simulink model "zumo_control_distance_heading"  (R2014a)
settings: Solver=ode3  SolverMode=SingleTasking  StartTime=0.0  StopTime=10  FixedStep=0.01  RelTol=1e-3
PreLoadFcn:
  | evalin('base','sim=1;');
  | evalin('base','control=0;');
  | prepareCurrentFolderForZumo;
  | load MagnetometerBus;
model workspace (MAT data in the model file):
  axleLength = Simulink.Parameter
  axleLength.Value = 9.8
  axleLength.Description = 'Distance between tire contact points
    | of the two wheels/treads
    | in units of centimeters.'
  axleLength.DataType = 'auto'
  commandPercmPerSecond = Simulink.Parameter
  commandPercmPerSecond.Value = 3.9547
  commandPercmPerSecond.Description = 'Convert units of ''command'' 
    | to units of ''cm/s''.
    | 
    | ''command'' is a value in the range [-256, 255].'
  commandPercmPerSecond.DataType = 'auto'
  symmetrizeMotors = Simulink.Parameter
  symmetrizeMotors.Value = 1
  symmetrizeMotors.Description = 'Scale one of the motor commands down 
    | (not up) to balance the motors. 
    | Once balanced, a value of x sent to either
    | motor will produce the same rate of rotation
    | in both motors.'
  symmetrizeMotors.DataType = 'auto'
  sampleTime = Simulink.Parameter
  sampleTime.Value = 0.01
  sampleTime.Description = 'Sample time (in seconds) of the trajectory simulator.'
  sampleTime.DataType = 'auto'
  commandThreshold = Simulink.Parameter
  commandThreshold.Value = 31.875
  commandThreshold.DataType = 'auto'
  lineThreshold = Simulink.Parameter
  lineThreshold.Value = 500
  lineThreshold.DataType = 'auto'
  velocity = Simulink.Parameter
  velocity.Value = 10
  velocity.Description = 'cm / s'
  velocity.DataType = 'auto'
  waveLength = Simulink.Parameter
  waveLength.Value = 8.6
  waveLength.Description = 'Units of cm.
    | 
    | The following condition must be satisfied: 
    | waveLength > 2*pi * velocity / sqrt(0.5 / sampleTime)
    | 
    | For reference,
    | robotLength = 8.6 cm
    | '
  waveLength.DataType = 'auto'
  compassBias = Simulink.Parameter
  compassBias.Value = 0
  compassBias.DataType = 'auto'
undefined symbols (not defined in the file or in its folder): DiscIntNeverNeededParam, magnitude
libraries: simulink x2, ZumoBotLib x2
settings Model: ExtModeTrigDuration=2  Creator=pkasseba  LastModifiedBy=sandip
settings OptimizationCC: OptimizeModelRefInitCode=on  LifeSpan=1
settings DebuggingCC: UnderspecifiedInitializationDetection=Classic  SolverPrmCheckMsg=none  StateNameClashWarn=warning
settings HardwareCC: ProdBitPerInt=16  ProdBitPerPointer=8  ProdIntDivRoundTo=Zero  ProdEndianess=LittleEndian  ProdWordSize=8  ProdHWDeviceType=Atmel->AVR
settings SFSimCC: SimParseCustomCode=off
settings RTWCC: SystemTargetFile=realtime.tlc  GenerateMakefile=off  TemplateMakefile=realtime.tmf  Description=Run on Target Hardware  RTWVerbose=off  ProcessScript=realtime_make_rtw_hook
settings STFCustomTargetCC: TargetLibSuffix=.a  GenerateSampleERTMain=on  ConcurrentExecutionCompliant=off  GeneratePreprocessorConditionals=Use local settings  ERTCustomFileBanners=on  SupportNonInlinedSFcns=off  SupportVariableSizeSignals=on  MATLABClassNameForMDSCustomization=Simulink.SoftwareTarget.ERTCustomization  GRTInterface=off  SystemTargetFile=realtime.tlc
settings ERTTargetCC: CombineOutputUpdateFcns=off  SupportContinuousTime=on  SupportVariableSizeSignals=on  ExtModeTransport=3  ExtModeMexFile=ext_serial_win32_comm  ExtModeMexArgs=0 1 9600  ERTSrcFileBannerTemplate=realtime_code_template.cgt  ERTHdrFileBannerTemplate=realtime_code_template.cgt  ERTDataSrcFileTemplate=realtime_code_template.cgt  ERTDataHdrFileTemplate=realtime_code_template.cgt  ERTCustomFileTemplate=realtime_file_process.tlc

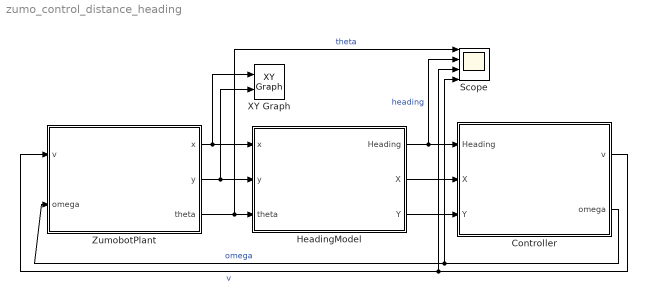
== system zumo_control_distance_heading ==
  Controller : Subsystem
  HeadingModel : Subsystem  Variant=on
  Scope : Scope  NumInputPorts=4
      settings: TimeRange=10  YMin=0~30.4~-1500~-5  YMax=375~33.6~1750~5  SaveName=ScopeData4
  XY Graph : simulink/Sinks/XY Graph  xmin=-20  xmax=20  ymin=-20  ymax=20  st=-1
  ZumobotPlant : Subsystem  Variant=on
  wires:
  Controller/1(v) -> Scope/3, ZumobotPlant/1(v)  "v"
  ZumobotPlant/1(x) -> XY Graph/1, HeadingModel/1(x)
  ZumobotPlant/2(y) -> XY Graph/2, HeadingModel/2(y)
  HeadingModel/1(Heading) -> Scope/2, Controller/1(Heading)  "heading"
  Controller/2(omega) -> Scope/4, ZumobotPlant/2(omega)  "omega"
  ZumobotPlant/3(theta) -> Scope/1, HeadingModel/3(theta)  "theta"
  HeadingModel/2(X) -> Controller/2(X)
  HeadingModel/3(Y) -> Controller/3(Y)

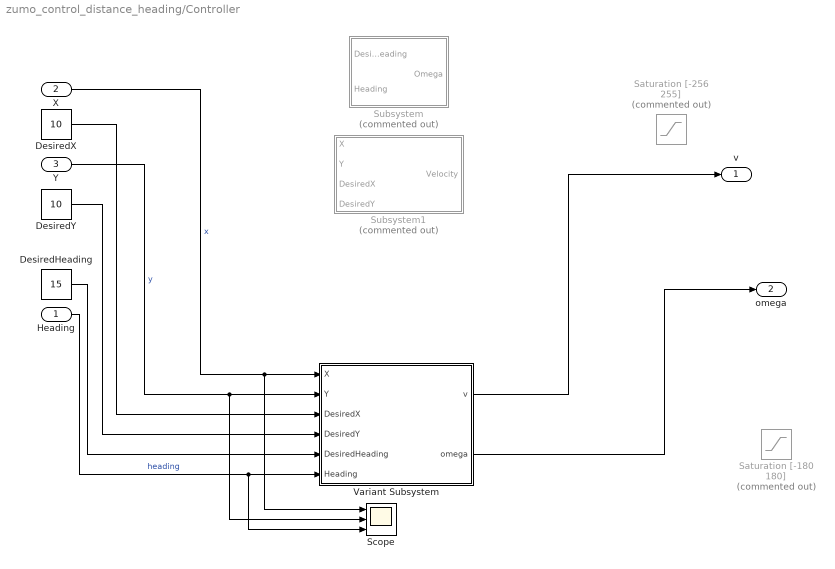
== system zumo_control_distance_heading/Controller ==
  Heading : Inport
  X : Inport  Port=2
  Y : Inport  Port=3
  DesiredHeading : Constant  Value=15
  DesiredX : Constant  Value=10
  DesiredY : Constant  Value=10
  Saturation [-180 180] : Saturate  Commented=on  UpperLimit=180  LowerLimit=-180
  Saturation [-256 255] : Saturate  Commented=on  UpperLimit=255  LowerLimit=-256
  Scope : Scope  NumInputPorts=3
      settings: YMin=0~-3~0  YMax=20~4~400  SaveName=ScopeData2
  Subsystem : Subsystem  Commented=on
  Subsystem1 : Subsystem  Commented=on
  Variant Subsystem : Subsystem  Variant=on  OverrideUsingVariant=control==0
  v : Outport
  omega : Outport  Port=2
  wires:
  X/1 -> Variant Subsystem/1(X), Scope/1  "x"
  Y/1 -> Variant Subsystem/2(Y), Scope/2  "y"
  DesiredX/1 -> Variant Subsystem/3(DesiredX)
  DesiredY/1 -> Variant Subsystem/4(DesiredY)
  DesiredHeading/1 -> Variant Subsystem/5(DesiredHeading)
  Heading/1 -> Variant Subsystem/6(Heading), Scope/3  "heading"
  Variant Subsystem/1(v) -> v/1
  Variant Subsystem/2(omega) -> omega/1

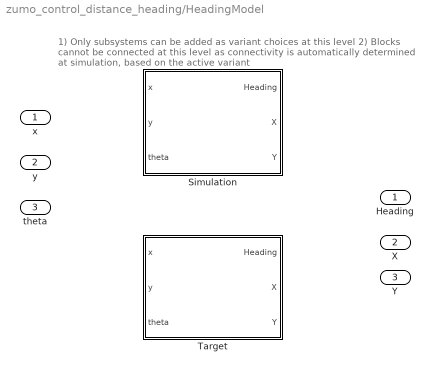
== system zumo_control_distance_heading/HeadingModel ==
  note: 1) Only subsystems can be added as variant choices at this level
      | 2) Blocks cannot be connected at this level as connectivity is
      | automatically determined at simulation, based on the active variant
  x : Inport
  y : Inport  Port=2
  theta : Inport  Port=3
  Simulation : Subsystem  VariantControl=sim==1
  Target : Subsystem  VariantControl=sim==0
  Heading : Outport
  X : Outport  Port=2
  Y : Outport  Port=3

== system zumo_control_distance_heading/ZumobotPlant ==
  note: 1) Only subsystems can be added as variant choices at this level
      | 2) Blocks cannot be connected at this level as connectivity is
      | automatically determined at simulation, based on the active variant
  v : Inport
  omega : Inport  Port=2
  Simulation : Subsystem  VariantControl=sim==1
  Target : Subsystem  VariantControl=sim==0
  x : Outport
  y : Outport  Port=2
  theta : Outport  Port=3

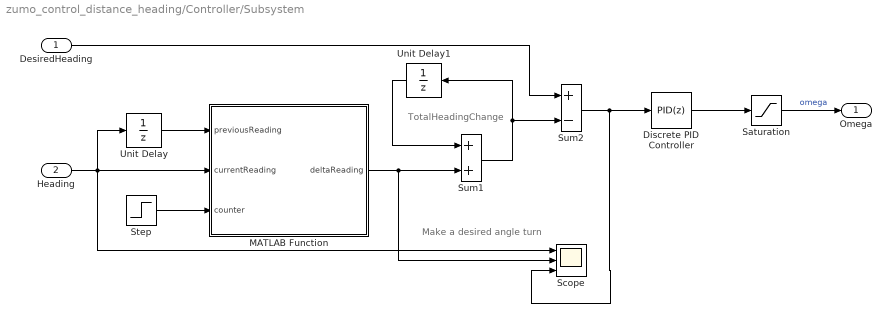
== system zumo_control_distance_heading/Controller/Subsystem ==
  note: Make a desired angle turn
  note: TotalHeadingChange
  DesiredHeading : Inport
  Heading : Inport  Port=2
  Discrete PID Controller : simulink/Continuous/PID Controller  Controller=PID  TimeDomain=Discrete-time  SampleTime=0.01  IntegratorMethod=Forward Euler  FilterMethod=Forward Euler  Form=Parallel  P=20  I=0  D=0  N=100  InitialConditionSource=internal  InitialConditionForIntegrator=0  InitialConditionForFilter=0  ExternalReset=none  LimitOutput=off  UpperSaturationLimit=inf  LowerSaturationLimit=-inf  LinearizeAsGain=off  AntiWindupMode=none  Kb=1  TrackingMode=off  Kt=1  PParamMin=[]  PParamMax=[]  IParamMin=[]  IParamMax=[]  DParamMin=[]  DParamMax=[]  NParamMin=[]  NParamMax=[]  KbParamMin=[]  KbParamMax=[]  KtParamMin=[]  KtParamMax=[]  POutMin=[]  POutMax=[]  IOutMin=[]  IOutMax=[]  DOutMin=[]  DOutMax=[]  NOutMin=[]  NOutMax=[]  KbOutMin=[]  KbOutMax=[]  KtOutMin=[]  KtOutMax=[]  IntegratorOutMin=[]  IntegratorOutMax=[]  FilterOutMin=[]  FilterOutMax=[]  SumOutMin=[]  SumOutMax=[]  SumI1OutMin=[]  SumI1OutMax=[]  SumI2OutMin=[]  SumI2OutMax=[]  SumI3OutMin=[]  SumI3OutMax=[]  SumDOutMin=[]  SumDOutMax=[]  SaturationOutMin=[]  SaturationOutMax=[]  IntegratorContinuousStateAttributes=''  IntegratorStateMustResolveToSignalObject=off  IntegratorRTWStateStorageClass=Auto  FilterContinuousStateAttributes=''  FilterStateMustResolveToSignalObject=off  FilterRTWStateStorageClass=Auto
  MATLAB Function : MATLAB Function  TreatAsAtomicUnit=on
  Saturation : Saturate  UpperLimit=200  LowerLimit=0
  Scope : Scope  NumInputPorts=3
      settings: YMin=266~-1~-4  YMax=266~1~-4
  Step : Step  Time=2*sampleTime  SampleTime=sampleTime
  Sum1 : Sum
  Sum2 : Sum  Inputs=+-
  Unit Delay : UnitDelay  SampleTime=-1
  Unit Delay1 : UnitDelay  SampleTime=-1
  Omega : Outport
  wires:
  Sum1/1 -> Unit Delay1/1, Sum2/2
  Step/1 -> MATLAB Function/3(counter)
  MATLAB Function/1(deltaReading) -> Scope/2, Sum1/2
  Sum2/1 -> Discrete PID Controller/1, Scope/3
  Saturation/1 -> Omega/1  "omega"
  Unit Delay/1 -> MATLAB Function/1(previousReading)
  Unit Delay1/1 -> Sum1/1
  DesiredHeading/1 -> Sum2/1
  Heading/1 -> Unit Delay/1, MATLAB Function/2(currentReading), Scope/1
  Discrete PID Controller/1 -> Saturation/1

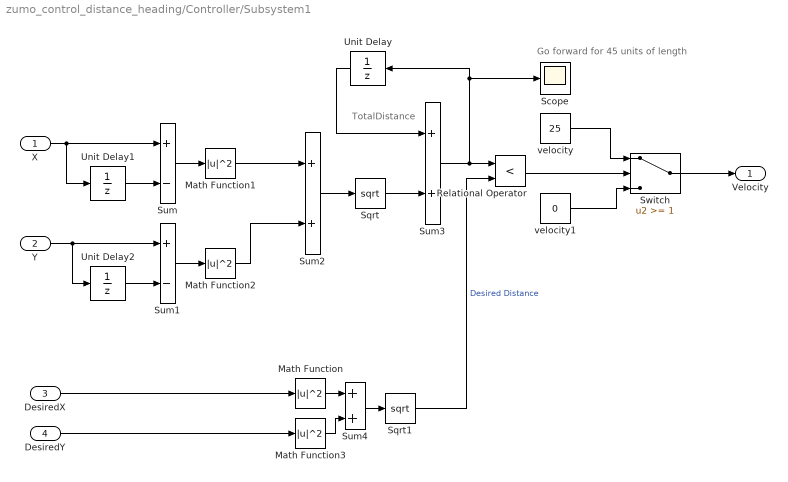
== system zumo_control_distance_heading/Controller/Subsystem1 ==
  note: Go forward for 45 units of length
  note: TotalDistance
  X : Inport
  Y : Inport  Port=2
  DesiredX : Inport  Port=3
  DesiredY : Inport  Port=4
  Math Function{,1..3} (4 alike) : Math  Operator=magnitude^2  SaturateOnIntegerOverflow=on
  Relational Operator : RelationalOperator  Operator=<  OutDataTypeStr=boolean
  Scope : Scope
      settings: YMin=0  YMax=50
  Sqrt : Sqrt  SaturateOnIntegerOverflow=on
  Sqrt1 : Sqrt  SaturateOnIntegerOverflow=on
  Sum : Sum  Inputs=+-
  Sum1 : Sum  Inputs=+-
  Sum2 : Sum
  Sum3 : Sum
  Sum4 : Sum
  Switch : Switch  Threshold=1
  Unit Delay : UnitDelay  SampleTime=-1
  Unit Delay1 : UnitDelay  SampleTime=-1
  Unit Delay2 : UnitDelay  SampleTime=-1
  velocity : Constant  Value=25
  velocity1 : Constant  Value=0
  Velocity : Outport
  wires:
  X/1 -> Unit Delay1/1, Sum/1
  Sqrt/1 -> Sum3/2
  Sum/1 -> Math Function1/1
  Sum2/1 -> Sqrt/1
  Math Function1/1 -> Sum2/1
  velocity/1 -> Switch/1
  Unit Delay1/1 -> Sum/2
  Math Function2/1 -> Sum2/2
  Switch/1 -> Velocity/1
  Sum1/1 -> Math Function2/1
  Unit Delay2/1 -> Sum1/2
  Y/1 -> Unit Delay2/1, Sum1/1
  Unit Delay/1 -> Sum3/1
  Sum3/1 -> Relational Operator/1, Scope/1, Unit Delay/1
  velocity1/1 -> Switch/3
  Relational Operator/1 -> Switch/2
  Math Function3/1 -> Sum4/2
  Math Function/1 -> Sum4/1
  Sum4/1 -> Sqrt1/1
  Sqrt1/1 -> Relational Operator/2  "Desired Distance"
  DesiredX/1 -> Math Function/1
  DesiredY/1 -> Math Function3/1

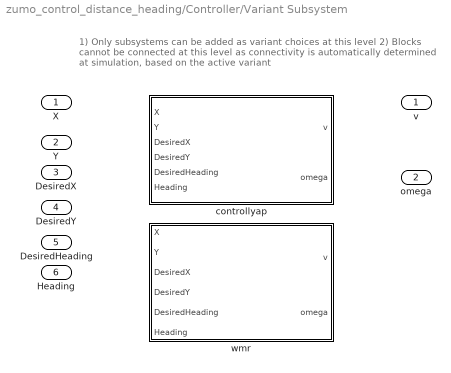
== system zumo_control_distance_heading/Controller/Variant Subsystem ==
  note: 1) Only subsystems can be added as variant choices at this level
      | 2) Blocks cannot be connected at this level as connectivity is
      | automatically determined at simulation, based on the active variant
  X : Inport
  Y : Inport  Port=2
  DesiredX : Inport  Port=3
  DesiredY : Inport  Port=4
  DesiredHeading : Inport  Port=5
  Heading : Inport  Port=6
  controllyap : MATLAB Function  TreatAsAtomicUnit=on  VariantControl=control==0
  wmr : MATLAB Function  TreatAsAtomicUnit=on  VariantControl=control==1
  v : Outport
  omega : Outport  Port=2

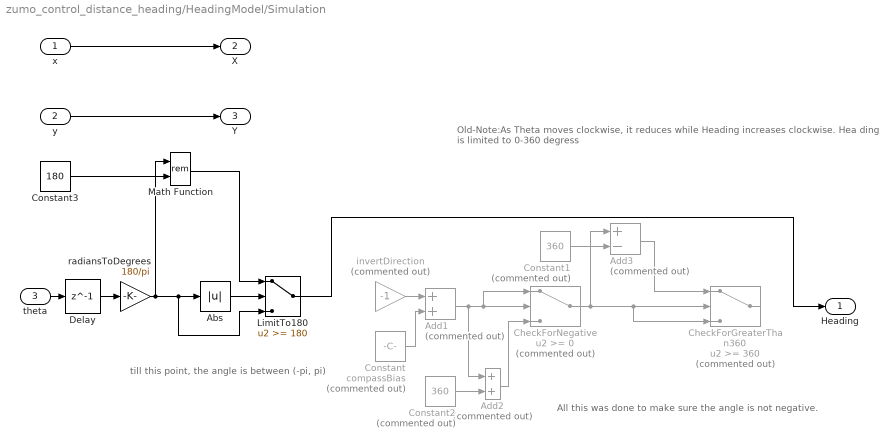
== system zumo_control_distance_heading/HeadingModel/Simulation ==
  note: till this point, the angle is between (-pi, pi)
  note: All this was done to make sure the angle is not negative.
  note: Old-Note:As Theta moves clockwise, it reduces while Heading increases clockwise.
      | Hea ding is limited to 0-360 degress
  x : Inport
  y : Inport  Port=2
  theta : Inport  Port=3
  Abs : Abs
  Add1 : Sum  Commented=on
  Add2 : Sum  Commented=on
  Add3 : Sum  Commented=on  Inputs=+-
  CheckForGreaterThan360 : Switch  Commented=on  Threshold=360
  CheckForNegative : Switch  Commented=on
  Constant : Constant  Commented=on  Value=compassBias
  Constant1 : Constant  Commented=on  Value=360
  Constant2 : Constant  Commented=on  Value=360
  Constant3 : Constant  Value=180
  Delay : Delay  DelayLength=1  InitialCondition=2*pi  SampleTime=sampleTime
  LimitTo180 : Switch  Threshold=180
  Math Function : Math  Operator=rem  SaturateOnIntegerOverflow=on
  invertDirection : Gain  Commented=on  Gain=-1
  radiansToDegrees : Gain  Gain=180/pi
  Heading : Outport
  X : Outport  Port=2
  Y : Outport  Port=3
  wires:
  x/1 -> X/1
  y/1 -> Y/1
  theta/1 -> Delay/1
  Delay/1 -> radiansToDegrees/1
  Constant/1 -> Add1/2
  Constant1/1 -> Add3/2
  Add3/1 -> CheckForGreaterThan360/1
  invertDirection/1 -> Add1/1
  Add1/1 -> Add2/1, CheckForNegative/2, CheckForNegative/1
  CheckForNegative/1 -> CheckForGreaterThan360/3, CheckForGreaterThan360/2, Add3/1
  Constant2/1 -> Add2/2
  Add2/1 -> CheckForNegative/3
  radiansToDegrees/1 -> Math Function/1, LimitTo180/3, Abs/1
  Constant3/1 -> Math Function/2
  Math Function/1 -> LimitTo180/1
  Abs/1 -> LimitTo180/2
  LimitTo180/1 -> Heading/1

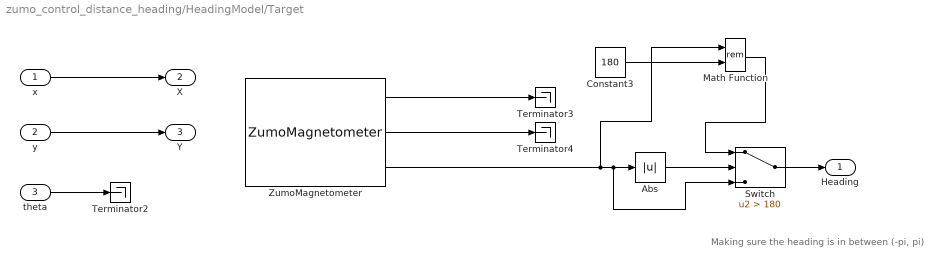
== system zumo_control_distance_heading/HeadingModel/Target ==
  note: Making sure the heading is in between (-pi, pi)
  x : Inport
  y : Inport  Port=2
  theta : Inport  Port=3
  Abs : Abs
  Constant3 : Constant  Value=180
  Math Function : Math  Operator=rem  SaturateOnIntegerOverflow=on
  Switch : Switch  Criteria=u2 > Threshold  Threshold=180
  Terminator2 : Terminator
  Terminator3 : Terminator
  Terminator4 : Terminator
  ZumoMagnetometer : ZumoBotLib/ZumoMagnetometer  sampletime_lsm=0.01  debug_lsm=on  minX_lsm=-512  maxX_lsm=-279  minY_lsm=-163  maxY_lsm=99  minZ_lsm=1302  maxZ_lsm=1580
      link override S-Function Builder: Parameters=sampletime_lsm,boolean(debug_lsm),minX_lsm,maxX_lsm,minY_lsm,maxY_lsm,minZ_lsm,boolean(maxZ_lsm)
  Heading : Outport
  X : Outport  Port=2
  Y : Outport  Port=3
  wires:
  x/1 -> X/1
  y/1 -> Y/1
  theta/1 -> Terminator2/1
  ZumoMagnetometer/1 -> Terminator3/1
  ZumoMagnetometer/2 -> Terminator4/1
  Switch/1 -> Heading/1
  Abs/1 -> Switch/2
  ZumoMagnetometer/3 -> Math Function/1, Switch/3, Abs/1
  Constant3/1 -> Math Function/2
  Math Function/1 -> Switch/1

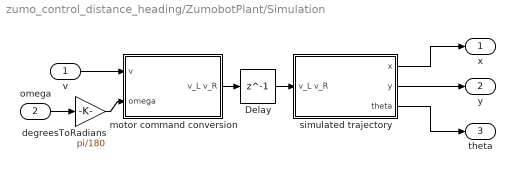
== system zumo_control_distance_heading/ZumobotPlant/Simulation ==
  v : Inport
  omega : Inport  Port=2
  Delay : Delay  DelayLength=1  InitialCondition=0
  degreesToRadians : Gain  Gain=pi/180
  motor command conversion : Subsystem
  simulated trajectory : Subsystem
  x : Outport
  y : Outport  Port=2
  theta : Outport  Port=3
  wires:
  v/1 -> motor command conversion/1(v)
  simulated trajectory/1(x) -> x/1
  simulated trajectory/2(y) -> y/1
  omega/1 -> degreesToRadians/1
  simulated trajectory/3(theta) -> theta/1
  degreesToRadians/1 -> motor command conversion/2(omega)
  motor command conversion/1(v_L v_R) -> Delay/1
  Delay/1 -> simulated trajectory/1(v_L v_R)

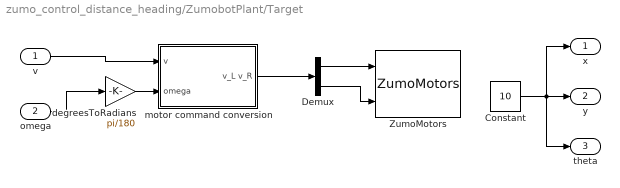
== system zumo_control_distance_heading/ZumobotPlant/Target ==
  v : Inport
  omega : Inport  Port=2
  Constant : Constant  Value=10
  Demux : Demux  Outputs=2
  ZumoMotors : ZumoBotLib/ZumoMotors  flipLeft=off  flipRight=off
  degreesToRadians : Gain  Gain=pi/180
  motor command conversion : Subsystem
  x : Outport
  y : Outport  Port=2
  theta : Outport  Port=3
  wires:
  motor command conversion/1(v_L v_R) -> Demux/1
  Demux/1 -> ZumoMotors/1
  Demux/2 -> ZumoMotors/2
  v/1 -> motor command conversion/1(v)
  Constant/1 -> theta/1, x/1, y/1
  omega/1 -> degreesToRadians/1
  degreesToRadians/1 -> motor command conversion/2(omega)

== system zumo_control_distance_heading/ZumobotPlant/Simulation/motor command conversion ==
  note: or in matrix notation,
  note: v_L  = v - omega * axleLength/2
      | v_R = v + omega * axleLength/2
  note: [v_L; v_R] = [1 -axleLength/2; 1 axleLength/2] * [v; omega]
  v : Inport
  omega : Inport  Port=2
  Mux : Mux  Inputs=2
  Saturation [-256 255] : Saturate  UpperLimit=255  LowerLimit=-256
  change parameters : Gain  Gain=[1 -axleLength/2; 1 axleLength/2]  Multiplication=Matrix(K*u)
  change units : Gain  Gain=commandPercmPerSecond
  symmetrize motors : Gain  Gain=[1 symmetrizeMotors]
  v_L v_R : Outport
  wires:
  change parameters/1 -> symmetrize motors/1  "v_L v_R"
  change units/1 -> Saturation [-256 255]/1  "v_L v_R (command)"
  symmetrize motors/1 -> change units/1  "v_L v_R (cm/s)"
  Saturation [-256 255]/1 -> v_L v_R/1
  Mux/1 -> change parameters/1
  omega/1 -> Mux/2
  v/1 -> Mux/1

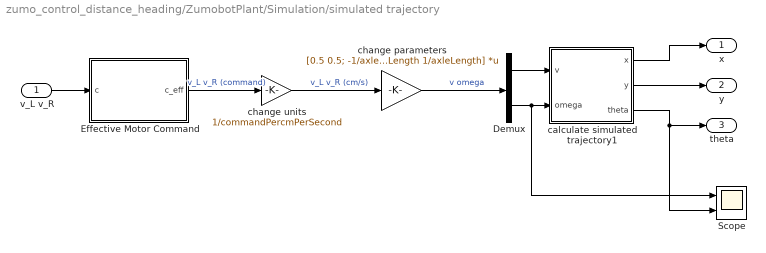
== system zumo_control_distance_heading/ZumobotPlant/Simulation/simulated trajectory ==
  v_L v_R : Inport
  Demux : Demux  Outputs=2
  Effective Motor Command : Subsystem
  Scope : Scope  NumInputPorts=2
      settings: YMin=-1~0.188496  YMax=1~0.188496  SaveName=ScopeData3
  calculate simulated trajectory1 : Subsystem
  change parameters : Gain  Gain=[0.5 0.5; -1/axleLength 1/axleLength]  Multiplication=Matrix(K*u)
  change units : Gain  Gain=1/commandPercmPerSecond
  x : Outport
  y : Outport  Port=2
  theta : Outport  Port=3
  wires:
  Demux/2 -> Scope/1, calculate simulated trajectory1/2(omega)
  Demux/1 -> calculate simulated trajectory1/1(v)
  v_L v_R/1 -> Effective Motor Command/1(c)
  Effective Motor Command/1(c_eff) -> change units/1  "v_L v_R (command)"
  change units/1 -> change parameters/1  "v_L v_R (cm/s)"
  change parameters/1 -> Demux/1  "v omega"
  calculate simulated trajectory1/2(y) -> y/1
  calculate simulated trajectory1/1(x) -> x/1
  calculate simulated trajectory1/3(theta) -> Scope/2, theta/1

== system zumo_control_distance_heading/ZumobotPlant/Target/motor command conversion ==
  note: or in matrix notation,
  note: v_L  = v - omega * axleLength/2
      | v_R = v + omega * axleLength/2
  note: [v_L; v_R] = [1 -axleLength/2; 1 axleLength/2] * [v; omega]
  v : Inport
  omega : Inport  Port=2
  Mux : Mux  Inputs=2
  Saturation [-256 255] : Saturate  UpperLimit=255  LowerLimit=-256
  change parameters : Gain  Gain=[1 -axleLength/2; 1 axleLength/2]  Multiplication=Matrix(K*u)
  change units : Gain  Gain=commandPercmPerSecond
  symmetrize motors : Gain  Gain=[1 symmetrizeMotors]
  v_L v_R : Outport
  wires:
  change parameters/1 -> symmetrize motors/1  "v_L v_R"
  change units/1 -> Saturation [-256 255]/1  "v_L v_R (command)"
  symmetrize motors/1 -> change units/1  "v_L v_R (cm/s)"
  Saturation [-256 255]/1 -> v_L v_R/1
  Mux/1 -> change parameters/1
  omega/1 -> Mux/2
  v/1 -> Mux/1

== system zumo_control_distance_heading/ZumobotPlant/Simulation/simulated trajectory/Effective Motor Command ==
  note: Zumobot does not move when given a command
      | with an abs less than 50 on a smooth surface,
      | so such commands are effectively 0.
  note: Do not saturate this signal.The process of symmetrizing
      | the motor commands gives rise to this artificial signal,
      | which can exceed the value of 255.
  c : Inport
  Abs : Abs
  Constant1 : Constant  Value=0
  Sum : Sum  Inputs=|+-
  Switch : Switch
  command threshold : Constant  Value=commandThreshold
  symmetrize motors : Gain  Gain=[1 1/symmetrizeMotors]
  c_eff : Outport
  wires:
  Switch/1 -> c_eff/1
  symmetrize motors/1 -> Abs/1, Switch/1
  Sum/1 -> Switch/2
  Abs/1 -> Sum/1
  command threshold/1 -> Sum/2
  c/1 -> symmetrize motors/1  "v_L v_R"
  Constant1/1 -> Switch/3

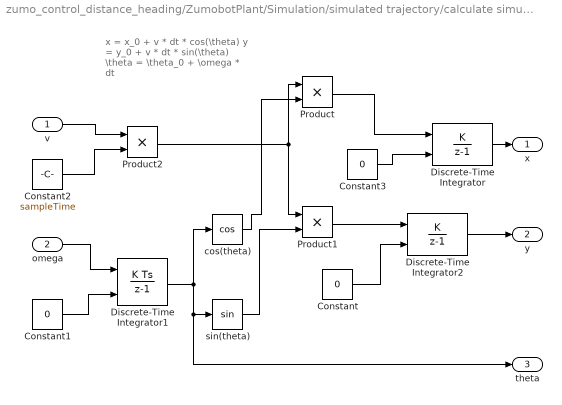
== system zumo_control_distance_heading/ZumobotPlant/Simulation/simulated trajectory/calculate simulated trajectory1 ==
  note: x = x_0 + v * dt * cos(\theta)
      | y = y_0 + v * dt * sin(\theta)
      | \theta = \theta_0 + \omega * dt
  v : Inport
  omega : Inport  Port=2
  Constant : Constant  Value=0
  Constant1 : Constant  Value=0
  Constant2 : Constant  Value=sampleTime
  Constant3 : Constant  Value=0
  Discrete-Time Integrator : DiscreteIntegrator  IntegratorMethod=Accumulation: Forward Euler  InitialConditionSource=external  InitialConditionSetting=State (most efficient)  SampleTime=-1  ICPrevOutput=DiscIntNeverNeededParam  ICPrevScaledInput=DiscIntNeverNeededParam
  Discrete-Time Integrator1 : DiscreteIntegrator  InitialConditionSource=external  SampleTime=-1  ICPrevOutput=DiscIntNeverNeededParam  ICPrevScaledInput=DiscIntNeverNeededParam
  Discrete-Time Integrator2 : DiscreteIntegrator  IntegratorMethod=Accumulation: Forward Euler  InitialConditionSource=external  InitialConditionSetting=State (most efficient)  SampleTime=-1  ICPrevOutput=DiscIntNeverNeededParam  ICPrevScaledInput=DiscIntNeverNeededParam
  Product : Product
  Product1 : Product
  Product2 : Product
  cos(theta) : Trigonometry  Operator=cos
  sin(theta) : Trigonometry
  x : Outport
  y : Outport  Port=2
  theta : Outport  Port=3
  wires:
  omega/1 -> Discrete-Time Integrator1/1
  v/1 -> Product2/1
  Discrete-Time Integrator1/1 -> theta/1, sin(theta)/1, cos(theta)/1
  Product/1 -> Discrete-Time Integrator/1
  cos(theta)/1 -> Product/2
  Product2/1 -> Product/1, Product1/1
  sin(theta)/1 -> Product1/2
  Constant3/1 -> Discrete-Time Integrator/2
  Constant1/1 -> Discrete-Time Integrator1/2
  Constant2/1 -> Product2/2
  Discrete-Time Integrator/1 -> x/1
  Product1/1 -> Discrete-Time Integrator2/1
  Discrete-Time Integrator2/1 -> y/1
  Constant/1 -> Discrete-Time Integrator2/2

== matlab function zumo_control_distance_heading/Controller/Subsystem/MATLAB Function ==
  data: previousReading input; deltaReading output; currentReading input; counter input
function deltaReading = handle360jump(previousReading, currentReading, counter)
%#codegen
deltaReading = 0;
if counter
    deltaReading = currentReading - previousReading;
    if abs(deltaReading) > 300
        if deltaReading > 0
            deltaReading = 360 - currentReading + previousReading;
        else
            deltaReading = 360 + deltaReading;
        end
    end
end
deltaReading = abs(deltaReading);

== matlab function zumo_control_distance_heading/Controller/Variant Subsystem/wmr ==
  data: X input; v output; Y input; DesiredX input; DesiredY input; DesiredHeading input; Heading input; omega output
function [v, omega] = wmr(X,Y,DesiredX,DesiredY,DesiredHeading, Heading)
%#codegen
% This function expects the dstates to be the difference of 
% dx = x_curr - x_dest; dy = y_curr - y_dest; dth = th_curr - th_dest;
persistent flag_initialize v_temp
if isempty(flag_initialize)
    flag_initialize = 1;
end
if isempty(v_temp)
    v_temp = 0;
end

dx = X - DesiredX;% cm
dy = Y - DesiredY;% cm
dth_degrees = Heading - DesiredHeading;% degrees (between 0 - 360)
dth = dth_degrees * pi/180; %in radians

dist_res = 1; %cm
heading_res = 5; %degrees
kp1 = 2;
kp2 = 12;
kd1 = 3;
kd2 = 7;
dt = 0.01;

if norm([dx dy]) < dist_res
    v = 0; %cm/s
    v_out = 0;
    if abs(dth_degrees) < heading_res
        omega = 0;%rad/s
    else
        omega = 360;%deg/s
    end
    %disp('Returning early.');
    return;
end
%% 
cth = cos(dth);
sth = sin(dth);

%% region division
region = 0; % initialize region
if dx >= 0 && dy >= 0     % add
    region = 1;
elseif dx < 0 && dy >= 0  % sugar
    region = 2;
elseif dx < 0 && dy < 0   % to
    region = 3;
elseif dx >= 0 && dy < 0  % coffee
    region = 4;
else
    error('Bad region: should not be here.');
end
%% region based inputs
if flag_initialize
    if region == 2 || region == 3
        v_temp = 32; %min threshold
    else % region = 1 || 4
        v_temp = -32; %min threshold
    end
    flag_initialize = 0;
end
% omega = 0;
%% computing v and omega 
v = v_temp;
v_out = v_temp;
xd = v*cth;
yd = v*sth;

u1 = -kp1*dx - kd1*xd;
u2 = -kp2*dy - kd2*yd;

v_temp = v_temp + (u1*cth + u2*sth) * dt; % cm/s
% v_prime = v_temp;
% saturate v_prime to a max of +255/-256 cm/s
% if v_prime > 255
%     v_prime = 255;
% elseif v_prime < -256
%     v_prime = -256;
% elseif v_prime < 32 && v_prime >= 0
%     v_prime = 32;
%     v_temp = v_prime;
% elseif v_prime > -32 && v_prime < 0
%     v_prime = -32;
%     v_temp = v_prime;
% end
v_tild = v_temp;
dvel = 5;
if abs(v_tild) < dvel
    v_tild = dvel;
%     v_temp = v_tild;
end

omega_rad_s = (u2*cth - u1*sth)/(v_tild); %rad/s

% convert rad/s into deg/s (as the plant model accepts that)
omega = omega_rad_s * (180/pi);

% % maximum omega(rad/s) allowed = ~2*pi/sec
% if omega > 360
%     omega= 360;
% elseif omega < -360
%     omega = -360;
% end

== matlab function zumo_control_distance_heading/Controller/Variant Subsystem/controllyap ==
  data: X input; v output; Y input; DesiredX input; DesiredY input; DesiredHeading input; Heading input; omega output
function [v, omega] = controllyap(X,Y,DesiredX,DesiredY,DesiredHeading,Heading)


dx =-(X - DesiredX);% cm
dy = -(Y - DesiredY);% cm
phi_des = DesiredHeading*pi/180;
phi_deg = Heading;
phi = phi_deg*pi/180;
%phi = Heading;
e = sqrt(dx^2+dy^2);

if e < 2
    v = 0;
    omega = 0;
    return;
end

% dir = [cos(phi_des),sin(phi_des)];
ang = atan2(sin(phi_des),cos(phi_des));
theta = atan2(dy,dx)-ang;
alpha = atan2(dy,dx)-phi;  
gamma = 1;
k = 1;
h = 1;
dist_res = .01; %cm
heading_res = 1; %degrees

omega = k*alpha+gamma*((cos(alpha)*sin(alpha))/alpha)*(alpha+h*theta);
v =  cos(alpha)*e*gamma;
omega = omega * (180/pi);
